simulink model "MCU_Simulation_Architecture"  (R2022b)
settings: Solver=FixedStepDiscrete  StartTime=0.0  StopTime=10  FixedStep=TimeSteps.ModelStep  RelTol=1e-6
PreLoadFcn:
  | addpath('tools');
  | addpath('tools\Config_UI');
  | addpath('tools\support');
  | addpath('tools\support\PlantModel');
  | addpath('tools\FMIKit_for_Simulink');
  | addpath('tools\SpeedCommand');
  | addpath('tools\SpeedCommand\exe');
  | addpath('tools\SpeedCommand\view');
  | addpath('tools\MciAPI');
  | addpath('tools\MciAPI\exe');
  | addpath('tools\MciAPI\exe\enums');
  | addpath('tools\Read_PDB_File');
  | addpath('tools\Read_PDB_File\exe');
  | addpath('tools\PILComm');
  | addpath('tools\PILComm\exe');
  | addpath('tools\CompileLink');
  | 
  | addpath('exe');
  | addpath('source');
  | addpath(genpath('plant_model'))
  | addpath(genpath('ParametersFiles'))
  | 
  | clear all;
  | 
  | try
  | FMIKit.initialize()
  | catch
  | display('FMI Kit Initialization Skipped');
  | end
  | 
  | Sim_Arch_Config_UI_App;
PostLoadFcn:
  | myws = get_param(gcs, 'modelworkspace');
  | myws.clear;
  | clear myws;
  | evalin('base', 'recompile_mcu_sim_arch = 1;');
  | updateModelWS(gcs);
  | 
  | variant_adc_out_mode = 0; % SIL Mode
  | 
  | ModelConfig_init_MCU_SimArch;
InitFcn:
  | if (evalin('base', 'exist(''smlarch_need_reset'') == 1'))
  |     msgbox('Reload Variables before Running');
  |     set_param(gcs, 'SimulationCommand', 'stop');
  | end
  | BusInit;
  | if(  (exist('SimArchUID')) && (strcmp(SimArchUID, 'a') == 1)  )
  |     updateModelWS(gcs);
  | end
  | useModelWS(gcs);
  | Simulink.sdi.close;
model workspace (MAT data in the model file):
  DC_Bus.Const_Vbus = 325
  InputCircuit.R_line = 0.8
  InputCircuit.L_line = 5e-05
  InputCircuit.C_buscap = 0.00022
  InputCircuit.R_diode = 0.068
  InputCircuit.R_buscap = 0.904
  InputCircuit.V_knee = 0.75
  InputCircuit.G_off = 1.25e-08
  InputCircuit.L_pfc = 0.0035
  InputCircuit.R_pfc = 0.45
  InputCircuit.Vr = 230
  InputCircuit.Vdc_i = 300
  InputCircuit.freq = 50
  InputCircuit.C1 = -0.200926
  InputCircuit.C2 = 1.64303
  InputCircuit.Cvolt = 0.00738585
  InputCircuit.Vcc = 3.3
  InputCircuit.ADCBit = 12
  InputCircuit.PGA_Gain = 1
  Mechanical.belt_ratio = 10
  Mechanical.JDrum = 0.0636792
  Mechanical.damp = 0.28
  Mechanical.m_unb = 0
  Mechanical.r_unb = 0.254
  Mechanical.M_D = 1
  Mechanical.M = 0.2
  Mechanical.R_Drum = 0.254
  Mechanical.R_J = 0.05
  Mechanical.CF = 0
  Motor.Electrical.Rs_a_Ref = 2.87
  Motor.Electrical.Rs_b_Ref = 2.87
  Motor.Electrical.Rs_c_Ref = 2.87
  Motor.Electrical.p_Pole_Pairs = 4
  Motor.Electrical.PM_Flux_f01 = 0.0845
  Motor.Electrical.PM_Flux_f02 = 0
  Motor.Electrical.PM_Flux_f03 = 0
  Motor.Electrical.PM_Flux_f04 = 0
  Motor.Electrical.PM_Flux_f05 = 0
  Motor.Electrical.PM_Flux_f06 = 0
  Motor.Electrical.PM_Flux_f07 = 0
  Motor.Electrical.PM_Flux_f08 = 0
  Motor.Electrical.PM_Flux_f09 = 0
  Motor.Electrical.PM_Flux_f10 = 0
  Motor.Electrical.PM_Flux_f11 = 0
  Motor.Electrical.PM_Flux_f12 = 0
  Motor.Electrical.PM_Flux_f13 = 0
  Motor.Electrical.ajust = 1.57
  Motor.Electrical.alpha_s = 0.004
  Motor.Mechanical.Jrotor = 0.000515
  Motor.Mechanical.B = 0
  Motor.Mechanical.Jadd = 0
  Motor.Mechanical.Rs_Temperature_Ref = 22
  Motor.Mechanical.PM_Temperature_Ref = 22
  Motor.Mechanical.TR = 11.4
  Motor.Power_Loss.Rot_Loss_Flag = 0
  Motor.Power_Loss.Rot_Loss_Speed0 = 0
  Motor.Power_Loss.Rot_Loss_Speed1 = 500
  Motor.Power_Loss.Rot_Loss_Speed2 = 3000
  Motor.Power_Loss.Rot_Loss_Speed3 = 4000
  Motor.Power_Loss.Rot_Loss_Speed4 = 5000
  Motor.Power_Loss.Rot_Loss_Speed5 = 7000
  Motor.Power_Loss.Rot_Loss_Speed6 = 12000
  Motor.Power_Loss.Rot_Loss_Speed7 = 18000
  Motor.Power_Loss.Rot_Loss_Power0 = 0
  Motor.Power_Loss.Rot_Loss_Power1 = 1
  Motor.Power_Loss.Rot_Loss_Power2 = 12
  Motor.Power_Loss.Rot_Loss_Power3 = 19
  Motor.Power_Loss.Rot_Loss_Power4 = 26
  Motor.Power_Loss.Rot_Loss_Power5 = 35
  Motor.Power_Loss.Rot_Loss_Power6 = 41
  Motor.Power_Loss.Rot_Loss_Power7 = 56
  Motor.Inductance_Variation.Ld_a0 = 0.02117
  Motor.Inductance_Variation.Ld_a1 = 0.02117
  Motor.Inductance_Variation.Ld_a2 = 0.02117
  Motor.Inductance_Variation.Ld_a3 = 0.02117
  Motor.Inductance_Variation.Ld_a4 = 0.02117
  Motor.Inductance_Variation.Ld_a5 = 0.02117
  Motor.Inductance_Variation.Ld_a6 = 0.02117
  Motor.Inductance_Variation.Ld_a7 = 0.02117
  Motor.Inductance_Variation.Lq_b0 = 0.02744
  Motor.Inductance_Variation.Lq_b1 = 0.02777
  Motor.Inductance_Variation.Lq_b2 = 0.02742
  Motor.Inductance_Variation.Lq_b3 = 0.02646
  Motor.Inductance_Variation.Lq_b4 = 0.02426
  Motor.Inductance_Variation.Lq_b5 = 0.02329
  Motor.Inductance_Variation.Lq_b6 = 0.02241
  Motor.Inductance_Variation.Lq_b7 = 0.02241
  Motor.Inductance_Variation.I_pk0 = 0
  Motor.Inductance_Variation.I_pk1 = 1
  Motor.Inductance_Variation.I_pk2 = 2
  Motor.Inductance_Variation.I_pk3 = 3
  Motor.Inductance_Variation.I_pk4 = 4
  Motor.Inductance_Variation.I_pk5 = 5
  Motor.Inductance_Variation.I_pk6 = 6
  Motor.Inductance_Variation.I_pk7 = 7
  Paths.complete_file_R = 'ParametersFiles\Board_Parameters\HVPS_230VPFC\WindyStripH40_AC230VPFC.xml'
  Paths.complete_file_M = 'ParametersFiles\Motor_Parameters\BPM\sBPM\BPM_Hefei_H27.xml'
  Paths.complete_file_mc = 'ParametersFiles\Mechanical_Parameters\HA\Mechanical_HA.xml'
  Paths.chosen_dir_M = 'ParametersFiles\Motor_Parameters\BPM\sBPM'
  Paths.Setting_File_Path = 'C:\Users\BEDNASA\Desktop\HA_sBPM_T95123402.bin'
  Paths.Root_Path = 'C:\Data\Nucleus_Dev\Windy_MCU_sBPM\source'
  Paths.Object_Path = ''
  Thermal.Tstator = 22
  Thermal.Trotor = 22
  TimeSteps.ModelStep = 6.25e-05
  TimeSteps.InputCircuitStep = 6.25e-05
  Variant_Input_Circuit = 4
  Variant_Motor = 4
  Variant_Motor_Control = 1
  Variant_Sensor = 0
  config.MCI_Sampling_Frequency = 'Set'
  config.rect_flag = 0
  config.const_dcbus_flag = 1
  config.Root_Path_flag = 'Source Selected'
  config.Motor_Control_Source = 'Set'
  config.Control_Layer = 'SIL'
  config.Fast_ADC_Initialization_Flag = 'Set'
  config.Skip_Motor_Moving_Handler_Flag = 'Set'
  config.BoardVariant = 'AC230VPFC'
  config.MotorVariant = 'BPM_Hefei_H27'
  config.MechanicalVariant = 'HA_Spin'
  config.Setting_File_Flag = 'Set'
undefined symbols (not defined in the file): sigbuilder_block, steps
CloseFcn:
  | rmpath('support');
  | rmpath('Compile Scripts');
  | rmpath(genpath('plant_models'))
  | rmpath(genpath('MciAPI'));
  | clc;
  | clear all;
settings Model: Creator=consul.marchionne  LastModifiedBy=BEDNASA
settings SolverCC: AlgebraicLoopSolver=TrustRegion
settings DataIOCC: LimitDataPoints=on  ReturnWorkspaceOutputs=off
settings OptimizationCC: LifeSpan=inf
settings DebuggingCC: SolverPrmCheckMsg=warning  UnconnectedInputMsg=warning  UnconnectedOutputMsg=warning  UnconnectedLineMsg=warning  SFUnexpectedBacktrackingDiag=warning  SFNoUnconditionalDefaultTransitionDiag=warning  SFExecutionAtInitializationDiag=none  SFMachineParentedDataDiag=warning  ArithmeticOperatorsInVariantConditions=warning
settings HardwareCC: ProdBitPerPointer=32  ProdBitPerSizeT=32  ProdBitPerPtrDiffT=32  ProdLargestAtomicFloat=None  ProdIntDivRoundTo=Undefined  ProdEndianess=Unspecified  ProdWordSize=32  ProdHWDeviceType=32-bit Generic
settings ModelReferenceCC: UpdateModelReferenceTargets=IfOutOfDate  ModelReferenceNumInstancesAllowed=Single  ModelReferenceMinAlgLoopOccurrences=on  PropagateSignalLabelsOutOfModel=off
settings SFSimCC: SimUseLocalCustomCode=off  CustomCodeUndefinedFunction=UseInterfaceOnly
settings RTWCC: RTWUseLocalCustomCode=off
settings CodeAppCC: StateflowObjectComments=on
settings GRTTargetCC: TargetLangStandard=C89/C90 (ANSI)
settings ConfigComp: CovMetricSettings=dw  CovSaveCumulativeToWorkspaceVar=on  CovSaveSingleToWorkspaceVar=on  CovExternalEMLEnable=off  CovSFcnEnable=off

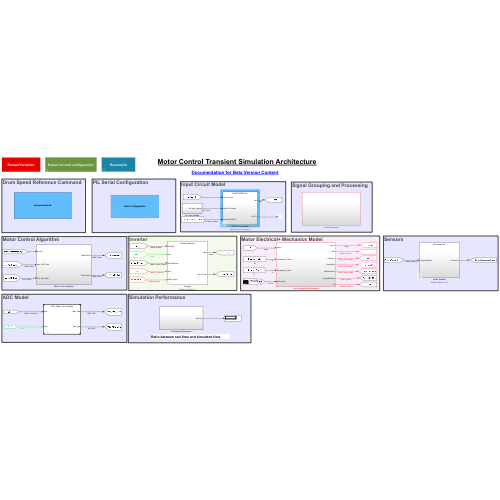
[thumbnail: Simulink's stored preview of the top-level diagram]
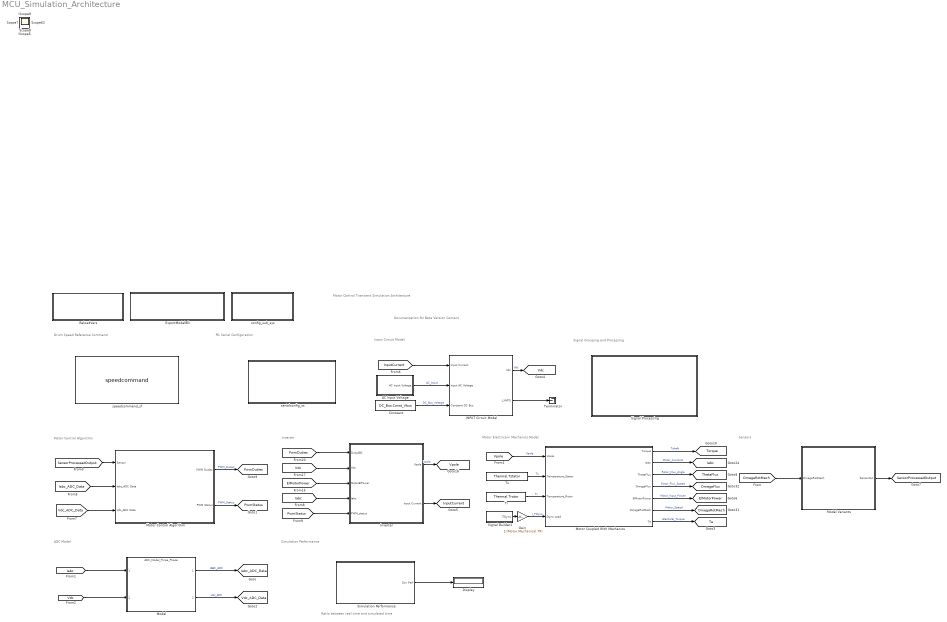
== system MCU_Simulation_Architecture ==
  note: Motor Control Transient Simulation Architecture
  note: Input Circuit Model
  note: Simulation Performance
  note: Ratio between real time and simulated time
  note: ADC Model
  note: Motor Electrical+ Mechanics Model
  note: Inverter
  note: Signal Grouping and Processing
  note: PIL Serial Configuration
  note: Motor Control Algorithm
  note: Sensors
  note: Drum Speed Reference Command
  note: Documentation for Beta Version Content
  AC Input Voltage : Subsystem
  Constant : Constant  Value=DC_Bus.Const_Vbus
  Display : Display
  ExportModelBlk : Subsystem  LoadFcn=|  mask{model_name=}
      | msk = Simulink.Mask.get(gcb);
      | bHandle = msk.getDialogControl('Control2');
      | bHandle.Enabled = 'on';
      | clear msk;
      | clear bHandle;
      mask prompts: model_name "Model's export name (no extension)"
      mask DialogControl Control2 Prompt: Export
      mask DialogControl Control2 Callback:
      | save_system('MCU_Simulation_Architecture');
      | if (strcmp(get_param(gcb, 'model_name'),'') == 1)
      |     msgbox('Must give a name to the model');
      | else
      |     exportSimArch(get_param(gcb, 'model_name'));
      | end
      mask Display: disp('Export current configuration');
  Gain : Gain  Gain=1/(Motor.Mechanical.TR)
  INPUT Circuit Model : Subsystem  Variant=on
      settings: AttributesFormatString=%<ActiveVariant>
  Inverter : Subsystem  Variant=on  mask(Inverter ideal){}
      mask help: Ideal model of 3-phase inverter
      settings: AttributesFormatString=%<ActiveVariant>
  Model : ModelReference  ModelNameDialog=ADC_Model_Three_Phase.slx  UsingDefaultArgumentValue=0,0,0,0,0,0,0,0,0,0,0,0  SimulationMode=Normal  ModelReferenceVersion=1.0  Gain_Iabc=InputCircuit.C1  Offset_Iabc=InputCircuit.C2  Vcc_Iabc=InputCircuit.Vcc  ADCBit_Iabc=InputCircuit.ADCBit  PGA_Gain_Iabc=1  Out_mode_Iabc=0  Gain_Vdc=InputCircuit.Cvolt  Offset_Vdc=0  Vcc_Vdc=InputCircuit.Vcc  ADCBit_Vdc=InputCircuit.ADCBit  PGA_Gain_Vdc=1  Out_mode_Vdc=0  SimulationMode=Normal
  Model Variants : Subsystem  Variant=on
      settings: AttributesFormatString=%<ActiveVariant>
  Motor Control Algorithm : Subsystem  SystemSampleTime=6.25e-5
  Motor Coupled With Mechanics : Subsystem  SystemSampleTime=0.000125
      settings: CopyFcn=|
      | blockname = gcb;
      |  linkstatus = lower(get_param(blockname,'LinkStatus'));
      | if strcmp(linkstatus,'resolved')
      |   set_param(gcb,'LinkStatus','none');
      | end
  ReloadVars : Subsystem
      settings: OpenFcn=|
      | evalin('base', 'clear smlarch_need_reset');
      | useModelWS(gcs);
      mask Display: disp('Reload Variables');
  Signal Builder1 : Subsystem  Tag=STV Subsys  LoadFcn=sigbuilder_block('load');  StartFcn=sigbuilder_block('start');  StopFcn=sigbuilder_block('stop');  ClipboardFcn=sigbuilder_block('clipboard');  mask(Sigbuilder block){tuvar=[0:10]}
      mask help: Simulink:masks:SigbuilderBlock_MD
      mask init:
      | if ~strcmp(get_param(bdroot(gcbh),'SimulationStatus'),'stopped') tuvar = sigbuilder_block('maskInit'); end
      settings: CopyFcn=sigbuilder_block('copy');  DeleteFcn=sigbuilder_block('delete');  ModelCloseFcn=sigbuilder_block('modelClose');  PreSaveFcn=sigbuilder_block('preSave');  PauseFcn=sigbuilder_block('pause');  ContinueFcn=sigbuilder_block('continue');  NameChangeFcn=sigbuilder_block('namechange');  OpenFcn=sigbuilder_block('open',[150 123 461.25 300 ]);  CloseFcn=sigbuilder_block('close');
      mask Display: plot(0, 0, 100, 100,[2, 2, 32, 32, 2], [68, 8, 8, 68, 68],[32, 2], [38, 38], [32, 19, 2],[53, 60, 44], [32, 17, 17, 2],[16, 16, 31, 31]);txt = getActiveGroup(gcbh);text(2, 100, txt,'verticalAlignment', 'top');
  Signal Processing : Subsystem
  Simulation Performance : Subsystem
  Terminator : Terminator
  Tr : Constant  Value=Thermal.Trotor
  Ts : Constant  Value=Thermal.Tstator
  config_sub_sys : Subsystem  TreatAsAtomicUnit=on  mask{mcu_recompile=on}
      mask prompts: mcu_recompile "Recompile"
      mask Display:
      | if (strcmp(get_param(gcb, 'mcu_recompile'),'off') == 1)
      |     disp('Do not Recompile');
      | else
      |     disp('Recompile');
      | end
  serialconfig_ss : Subsystem  mask{comdevtype=RS232, com_port=COM4, baudrate=57600}
      mask prompts: comdevtype "COM Type"; com_port "COM Port"
      mask TypeOptions comdevtype: RS232 | SPI
      mask Callback comdevtype:
      | maskStr = get_param(gcb,'comdevtype');
      | if strcmp(maskStr,'SPI')
      |     assignin('base', 'VARIANT_PIL_COMM', 2);
      | else
      |     assignin('base', 'VARIANT_PIL_COMM', 1);
      | end
      | clear maskStr;
      mask TypeOptions com_port: COM3 | COM4
      mask TypeOptions baudrate: 2400 | 4800 | 9600 | 19200 | 28800 | 38400 | 57600 | 115200 | 230400
      mask DialogControl ParameterGroupVar Prompt: RS232 Settings
      mask DialogControl rfrsh_button Prompt: Refresh Ports
      mask DialogControl rfrsh_button Callback:
      | devices = winqueryreg('name', 'HKEY_LOCAL_MACHINE', 'HARDWARE\DEVICEMAP\SERIALCOMM');
      | if (isempty(devices))
      |     com{1} = 'NONE';
      | else
      |     com = cell(1, length(devices));
      |    % h = waitbar(0,'Scanning Serial Ports...','Name','Scanning Serial Ports...');
      |     for i = 1:length(devices)
      |         com{i} = winqueryreg('HKEY_LOCAL_MACHINE', 'HARDWARE\DEVICEMAP\SERIALCOMM', devices{i});
      |     %    waitbar(i/length(devices),h);
      |     end
      | end
      | 
      | msk = Simulink.Mask.get(gcb);
      | p = msk.Parameters;
      | p(2).TypeOptions = com;
      | clear msk;
      | clear p;
      | clear com;
      | clear devices;
      mask Display: disp('Serial Configuration');
  speedcommand_sf : S-Function  InitFcn=|  StopFcn=|  FunctionName=speedcommand  Parameters=steps, Variant_Motor_Control  SFunctionDeploymentMode=off  EnableBusSupport=off
      InitFcn=|
      | transmission = evalin('base','Motor.Mechanical.TR');
      | if isempty(get_param(gcb,'UserData'))
      | steps = [];
      | else
      |     ud = get_param(gcb,'UserData');
      |     [pts,steps] = GenPlotCmds(ud.table);
      |     for i = 1:size(steps,1)
      |         steps(i,1) = steps(i,1) * transmission;
      |         steps(i,2) = steps(i,2) * transmission;
      |     end
      | end
      | clear transmission;
      | clear i;
      | clear ud;
      StopFcn=|
      | clear steps;
      | clear pts;
      settings: OpenFcn=SpeedCommandView;
  Scope{,2..12} (12 alike) : Scope
  tag scope: ElMotorPower=global, Iabc=global, Iabc_ADC_Data=global, InputCurrent=global, OmegaFlux=global, OmegaRotMech=global, PwmDuties=global, PwmStatus=global, SensorProcessedOutput=global, Te=global, ThetaFlux=global, Torque=global, Vdc=global, Vdc_ADC_Data=global, Vpole=global
  wires:
  Simulation Performance/1(Sim Perf) -> Display/1
  [Vpole] -> Motor Coupled With Mechanics/1(Vpole)  "Vpole"
  Motor Coupled With Mechanics/1(Torque) -> [Torque]  "Tshaft"
  Motor Coupled With Mechanics/2(Iabc) -> [Iabc]  "Motor_Currents"
  Motor Coupled With Mechanics/3(ThetaFlux) -> [ThetaFlux]  "Rotor_Flux_Angle"
  Motor Coupled With Mechanics/4(OmegaFlux) -> [OmegaFlux]  "Rotor_Flux_Speed"
  Motor Coupled With Mechanics/5(ElMotorPower) -> [ElMotorPower]  "Motor_Input_Power"
  Motor Coupled With Mechanics/6(OmegaRotMech) -> [OmegaRotMech]  "Motor_Speed"
  Motor Control Algorithm/1(PWM Duties) -> [PwmDuties]  "PWM_Duties"
  Motor Control Algorithm/2(PWM Status) -> [PwmStatus]  "PWM_Status"
  [SensorProcessedOutput] -> Motor Control Algorithm/1(Sensor)
  [Vdc] -> Model/2
  [Iabc] -> Model/1
  [Iabc_ADC_Data] -> Motor Control Algorithm/2(Iabc_ADC Data)
  Model/1 -> [Iabc_ADC_Data]  "IABC_ADC"
  Model/2 -> [Vdc_ADC_Data]  "Vdc_ADC"
  [Vdc_ADC_Data] -> Motor Control Algorithm/3(Vdc_ADC Data)
  Ts/1 -> Motor Coupled With Mechanics/2(Temperature_Stator)  "Ts"
  Tr/1 -> Motor Coupled With Mechanics/3(Temperature_Rotor)  "Tr"
  Gain/1 -> Motor Coupled With Mechanics/4(Dyno Load)  "i_TDyno"
  Signal Builder1/1(iTDyno) -> Gain/1
  Motor Coupled With Mechanics/7(Te) -> [Te]  "Electrical_Torque"
  [InputCurrent] -> INPUT Circuit Model/1(Input Current)
  AC Input Voltage/1(AC Input Voltage) -> INPUT Circuit Model/2(Input AC Voltage)  "AC_Input"
  Constant/1 -> INPUT Circuit Model/3(Constant DC Bus)  "DC_Bus_Voltage"
  INPUT Circuit Model/1(Vdc) -> [Vdc]  "Vdc"
  [PwmDuties] -> Inverter/1(DutyABC)
  [Vdc] -> Inverter/2(Vdc)
  [ElMotorPower] -> Inverter/3(MotorElPower)
  [Iabc] -> Inverter/4(Iabc)
  [PwmStatus] -> Inverter/5(PWM_status)
  Inverter/1(Vpole) -> [Vpole]  "Vpole"
  Inverter/2(Input Current) -> [InputCurrent]
  [OmegaRotMech] -> Model Variants/1(OmegaRotMech)
  Model Variants/1(SensorOut) -> [SensorProcessedOutput]
  INPUT Circuit Model/2(I_HVPS) -> Terminator/1

== system MCU_Simulation_Architecture/AC Input Voltage ==
  Sine Wave : Sin  Amplitude=InputCircuit.Vr*sqrt(2)  Frequency=InputCircuit.freq*2*pi
  AC Input Voltage : Outport  VectorParamsAs1DForOutWhenUnconnected=off
  wires:
  Sine Wave/1 -> AC Input Voltage/1

== system MCU_Simulation_Architecture/ExportModelBlk ==

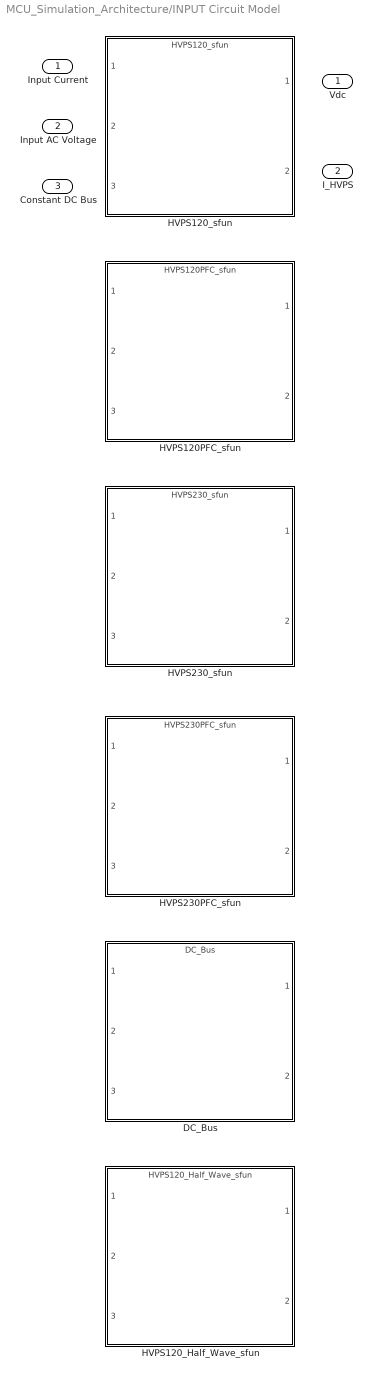
== system MCU_Simulation_Architecture/INPUT Circuit Model ==
  Input Current : Inport
  Input AC Voltage : Inport  Port=2
  Constant DC Bus : Inport  Port=3
  DC_Bus : ModelReference  ModelNameDialog=DC_Bus.slx  SimulationMode=Normal  VariantControl=Variant_Input_Circuit==5  ModelReferenceVersion=10.0
      settings: AttributesFormatString=%<ActiveVariant>
  HVPS120PFC_sfun : ModelReference  ModelNameDialog=HVPS120PFC_sfun.slx  SimulationMode=Normal  VariantControl=Variant_Input_Circuit==2  ModelReferenceVersion=10.4
      settings: AttributesFormatString=%<ActiveVariant>
  HVPS120_Half_Wave_sfun : ModelReference  ModelNameDialog=HVPS120_Half_Wave_sfun.slx  SimulationMode=Normal  VariantControl=Variant_Input_Circuit==6  ModelReferenceVersion=10.6
      settings: AttributesFormatString=%<ActiveVariant>
  HVPS120_sfun : ModelReference  ModelNameDialog=HVPS120_sfun.slx  SimulationMode=Normal  VariantControl=Variant_Input_Circuit==1  ModelReferenceVersion=10.8
      settings: AttributesFormatString=%<ActiveVariant>
  HVPS230PFC_sfun : ModelReference  ModelNameDialog=HVPS230PFC_sfun.slx  SimulationMode=Normal  VariantControl=Variant_Input_Circuit==4  ModelReferenceVersion=10.16
      settings: AttributesFormatString=%<ActiveVariant>
  HVPS230_sfun : ModelReference  ModelNameDialog=HVPS230_sfun.slx  SimulationMode=Normal  VariantControl=Variant_Input_Circuit==3  ModelReferenceVersion=10.3
      settings: AttributesFormatString=%<ActiveVariant>
  Vdc : Outport
  I_HVPS : Outport  Port=2

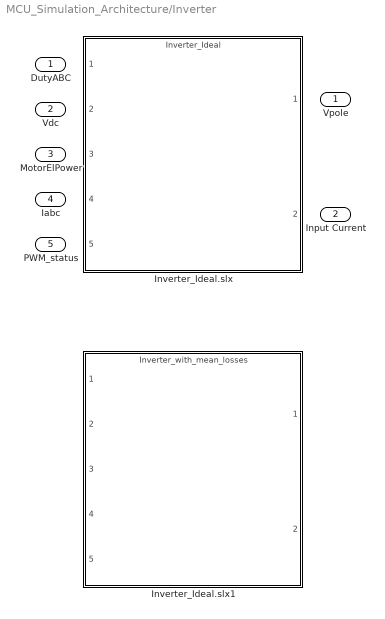
== system MCU_Simulation_Architecture/Inverter ==
  DutyABC : Inport  OutDataTypeStr=Bus: XabcBus
  Vdc : Inport  Port=2
  MotorElPower : Inport  Port=3
  Iabc : Inport  Port=4  OutDataTypeStr=Bus: XabcBus
  PWM_status : Inport  Port=5
  Inverter_Ideal.slx : ModelReference  ModelNameDialog=Inverter_Ideal.slx  SimulationMode=Normal  VariantControl=Variant_Inverter==1  OverrideUsingVariant=Variant1  ModelReferenceVersion=1.19  SimulationMode=Normal
      settings: AttributesFormatString=%<ActiveVariant>
  Inverter_Ideal.slx1 : ModelReference  ModelNameDialog=Inverter_with_mean_losses.slx  SimulationMode=Normal  VariantControl=Variant_Inverter==2  OverrideUsingVariant=Variant1  ModelReferenceVersion=10.27
      settings: AttributesFormatString=%<ActiveVariant>
  Vpole : Outport  OutDataTypeStr=Bus: XabcBus
  Input Current : Outport  Port=2

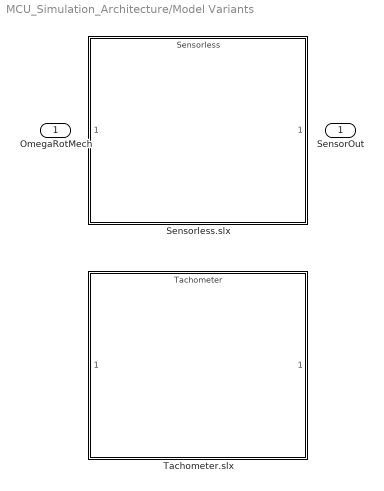
== system MCU_Simulation_Architecture/Model Variants ==
  OmegaRotMech : Inport
  Sensorless.slx : ModelReference  ModelNameDialog=Sensorless.slx  SimulationMode=Normal  VariantControl=Variant_Sensor == 0  ModelReferenceVersion=1.8
      settings: AttributesFormatString=%<ActiveVariant>
  Tachometer.slx : ModelReference  ModelNameDialog=Tachometer.slx  SimulationMode=Normal  VariantControl=Variant_Sensor == 1  ModelReferenceVersion=1.34
      settings: AttributesFormatString=%<ActiveVariant>
  SensorOut : Outport

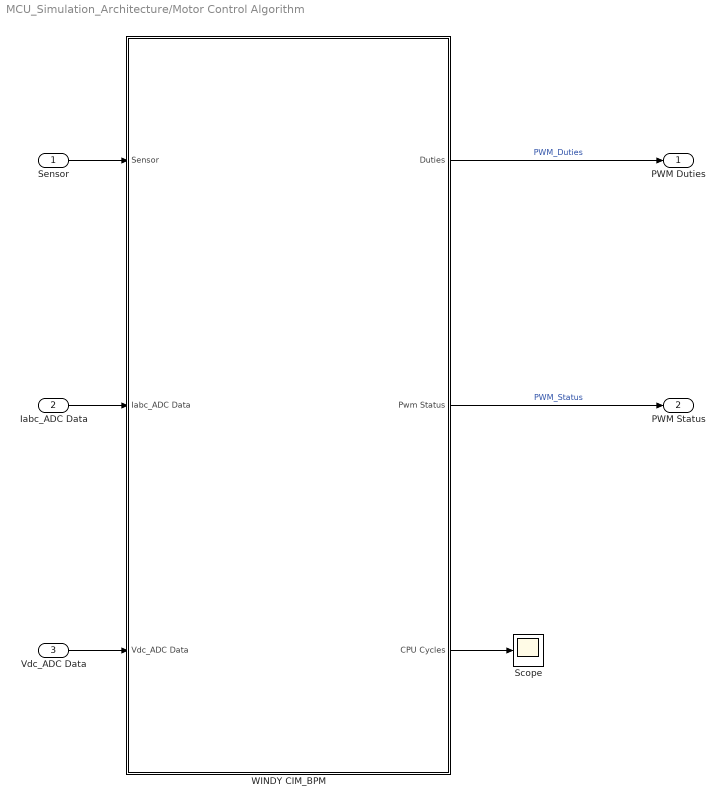
== system MCU_Simulation_Architecture/Motor Control Algorithm ==
  Sensor : Inport
  Iabc_ADC Data : Inport  Port=2
  Vdc_ADC Data : Inport  Port=3
  Scope : Scope
  WINDY CIM_BPM : Subsystem  Variant=on
  PWM Duties : Outport  VectorParamsAs1DForOutWhenUnconnected=off
  PWM Status : Outport  Port=2  VectorParamsAs1DForOutWhenUnconnected=off
  wires:
  WINDY CIM_BPM/1(Duties) -> PWM Duties/1  "PWM_Duties"
  WINDY CIM_BPM/2(Pwm Status) -> PWM Status/1  "PWM_Status"
  Sensor/1 -> WINDY CIM_BPM/1(Sensor)
  Iabc_ADC Data/1 -> WINDY CIM_BPM/2(Iabc_ADC Data)
  Vdc_ADC Data/1 -> WINDY CIM_BPM/3(Vdc_ADC Data)
  WINDY CIM_BPM/3(CPU Cycles) -> Scope/1

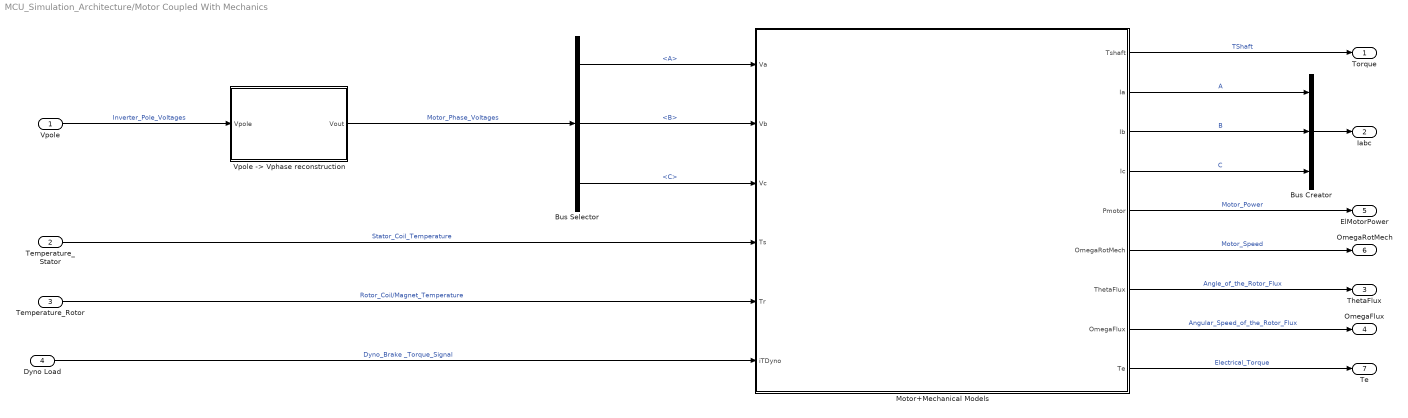
== system MCU_Simulation_Architecture/Motor Coupled With Mechanics ==
  Vpole : Inport  OutDataTypeStr=Bus: XabcBus
  Temperature_Stator : Inport  Port=2
  Temperature_Rotor : Inport  Port=3
  Dyno Load : Inport  Port=4
  Bus Creator : BusCreator  Inputs=3
  Bus Selector : BusSelector  OutputSignals=A,B,C
  Motor+Mechanical Models : Subsystem  Variant=on
      settings: AttributesFormatString=%<ActiveVariant>
  "Vpole -> Vphase reconstruction" : MATLAB Function  TreatAsAtomicUnit=on
  Torque : Outport  VectorParamsAs1DForOutWhenUnconnected=off
  Iabc : Outport  Port=2  OutDataTypeStr=Bus: XabcBus  VectorParamsAs1DForOutWhenUnconnected=off
  ThetaFlux : Outport  Port=3  VectorParamsAs1DForOutWhenUnconnected=off
  OmegaFlux : Outport  Port=4  VectorParamsAs1DForOutWhenUnconnected=off
  ElMotorPower : Outport  Port=5  VectorParamsAs1DForOutWhenUnconnected=off
  OmegaRotMech : Outport  Port=6  VectorParamsAs1DForOutWhenUnconnected=off
  Te : Outport  Port=7  VectorParamsAs1DForOutWhenUnconnected=off
  wires:
  Bus Creator/1 -> Iabc/1
  Vpole/1 -> "Vpole -> Vphase reconstruction"/1(Vpole)  "Inverter_Pole_Voltages"
  "Vpole -> Vphase reconstruction"/1(Vout) -> Bus Selector/1  "Motor_Phase_Voltages"
  Bus Selector/1 -> Motor+Mechanical Models/1(Va)  "<A>"
  Bus Selector/2 -> Motor+Mechanical Models/2(Vb)  "<B>"
  Bus Selector/3 -> Motor+Mechanical Models/3(Vc)  "<C>"
  Temperature_Stator/1 -> Motor+Mechanical Models/4(Ts)  "Stator_Coil_Temperature"
  Temperature_Rotor/1 -> Motor+Mechanical Models/5(Tr)  "Rotor_Coil/Magnet_Temperature"
  Dyno Load/1 -> Motor+Mechanical Models/6(iTDyno)  "Dyno_Brake _Torque_Signal"
  Motor+Mechanical Models/1(Tshaft) -> Torque/1  "TShaft"
  Motor+Mechanical Models/2(Ia) -> Bus Creator/1  "A"
  Motor+Mechanical Models/3(Ib) -> Bus Creator/2  "B"
  Motor+Mechanical Models/4(Ic) -> Bus Creator/3  "C"
  Motor+Mechanical Models/5(Pmotor) -> ElMotorPower/1  "Motor_Power"
  Motor+Mechanical Models/6(OmegaRotMech) -> OmegaRotMech/1  "Motor_Speed"
  Motor+Mechanical Models/7(ThetaFlux) -> ThetaFlux/1  "Angle_of_the_Rotor_Flux"
  Motor+Mechanical Models/8(OmegaFlux) -> OmegaFlux/1  "Angular_Speed_of_the_Rotor_Flux"
  Motor+Mechanical Models/9(Te) -> Te/1  "Electrical_Torque"

== system MCU_Simulation_Architecture/ReloadVars ==

== system MCU_Simulation_Architecture/Signal Builder1 ==
  Demux : Demux  Tag=STV Demux  Outputs=1
      settings: DisplayOption=none
  FromWs : FromWorkspace  Tag=STV FromWs  VariableName=tuvar
      SigBuilderData=|
      | common.afterFinalStr = 'Extrapolate'
      | common.sampleTime = 0
      | dataSet.timeRange = [0 30]
      | dataSet.name = 'Dyno_Load_Profile'
      | sbobj.Groups.Name = 'Dyno_Load_Profile'
      | sbobj.Groups.Signals.Name = 'iTDyno'
      | sbobj.Groups.Signals.XData = [0 0.8 4 20 28 30]
      | sbobj.Groups.Signals.YData = [0 0 0 0 0 0]
      | sbobj.Groups.TimeRange = [0 30]
  iTDyno : Outport  Tag=STV Outport  VectorParamsAs1DForOutWhenUnconnected=off
  wires:
  Demux/1 -> iTDyno/1
  FromWs/1 -> Demux/1

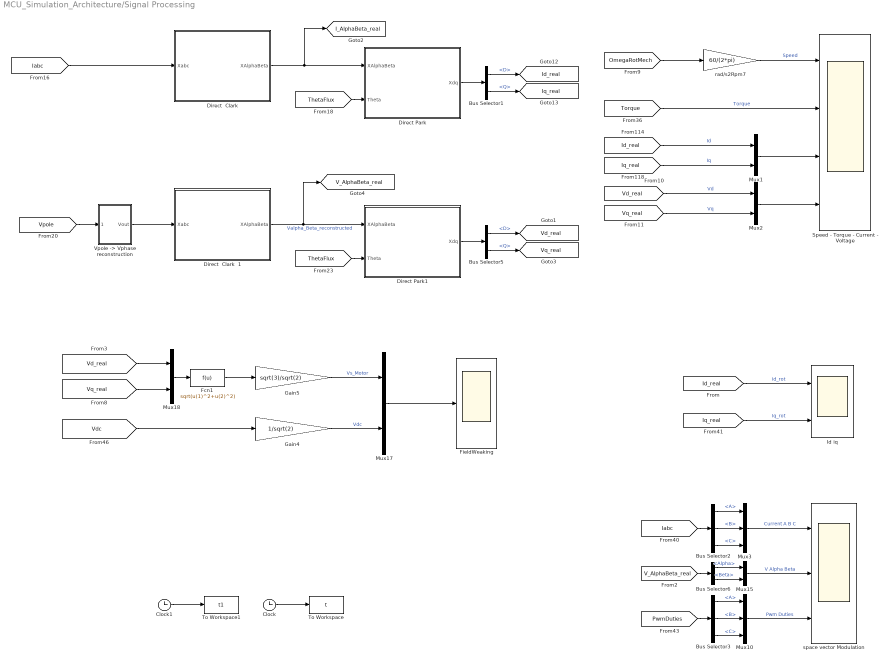
== system MCU_Simulation_Architecture/Signal Processing ==
  Bus Selector1 : BusSelector  OutputSignals=D,Q
  Bus Selector2 : BusSelector  OutputSignals=A,B,C
  Bus Selector3 : BusSelector  OutputSignals=A,B,C
  Bus Selector5 : BusSelector  OutputSignals=D,Q
  Bus Selector6 : BusSelector  OutputSignals=Alpha,Beta
  Clock : Clock
  Clock1 : Clock
  "Direct  Clark  " : MATLAB Function  TreatAsAtomicUnit=on  SystemSampleTime=SystemSampleTime  mask{SystemSampleTime=-1}
      mask prompts: SystemSampleTime "Simulink:blkprm_prompts:AllBlksSampleTime"
  Direct  Clark  1 : MATLAB Function  TreatAsAtomicUnit=on  SystemSampleTime=SystemSampleTime  mask{SystemSampleTime=-1}
      mask prompts: SystemSampleTime "Simulink:blkprm_prompts:AllBlksSampleTime"
  Direct Park : MATLAB Function  TreatAsAtomicUnit=on  SystemSampleTime=SystemSampleTime  mask{SystemSampleTime=-1}
      mask prompts: SystemSampleTime "Simulink:blkprm_prompts:AllBlksSampleTime"
  Direct Park1 : MATLAB Function  TreatAsAtomicUnit=on  SystemSampleTime=SystemSampleTime  mask{SystemSampleTime=-1}
      mask prompts: SystemSampleTime "Simulink:blkprm_prompts:AllBlksSampleTime"
  Fcn1 : Fcn  Expr=sqrt(u(1)^2+u(2)^2)
  "FieldWeaking " : Scope
  Gain4 : Gain  Gain=1/sqrt(2)
  Gain5 : Gain  Gain=sqrt(3)/sqrt(2)
  Id iq : Scope  NumInputPorts=2
  Mux{1..2,15,17..18} (5 alike) : Mux  Inputs=2
  Mux10 : Mux  Inputs=3
  Mux3 : Mux  Inputs=3
  Speed - Torque - Current - Voltage : Scope  NumInputPorts=4
  To Workspace : ToWorkspace  VariableName=t  SampleTime=-1
      settings: Save2DSignal=2-D array (concatenate along first dimension)
  To Workspace1 : ToWorkspace  VariableName=t1  SampleTime=-1
      settings: Save2DSignal=2-D array (concatenate along first dimension)
  "Vpole -> Vphase reconstruction" : MATLAB Function  TreatAsAtomicUnit=on
  rad/s2Rpm7 : Gain  Gain=60/(2*pi)
  space vector Modulation : Scope  NumInputPorts=3
  tag scope: I_AlphaBeta_real=global, Id_real=global, Iq_real=global, V_AlphaBeta_real=global, Vd_real=global, Vq_real=global
  wires:
  [OmegaRotMech] -> rad/s2Rpm7/1
  rad/s2Rpm7/1 -> Speed - Torque - Current - Voltage/1  "Speed"
  [Vq_real] -> Mux2/2  "Vq"
  [Id_real] -> Mux1/1  "Id"
  [Iabc] -> "Direct  Clark  "/1(Xabc)
  Direct Park/1(Xdq) -> Bus Selector1/1
  Bus Selector1/1 -> [Id_real]  "<D>"
  Bus Selector1/2 -> [Iq_real]  "<Q>"
  Fcn1/1 -> Gain5/1
  Mux18/1 -> Fcn1/1
  [Vd_real] -> Mux18/1
  [Vq_real] -> Mux18/2
  Mux17/1 -> "FieldWeaking "/1
  [Vdc] -> Gain4/1
  Bus Selector3/1 -> Mux10/1  "<A>"
  Bus Selector3/2 -> Mux10/2  "<B>"
  Bus Selector3/3 -> Mux10/3  "<C>"
  Mux10/1 -> space vector Modulation/3  "Pwm Duties"
  Bus Selector2/1 -> Mux3/1  "<A>"
  Bus Selector2/2 -> Mux3/2  "<B>"
  Bus Selector2/3 -> Mux3/3  "<C>"
  [Iabc] -> Bus Selector2/1
  [PwmDuties] -> Bus Selector3/1
  "Direct  Clark  "/1(XAlphaBeta) -> [I_AlphaBeta_real], Direct Park/1(XAlphaBeta)
  Clock/1 -> To Workspace/1
  Clock1/1 -> To Workspace1/1
  [Id_real] -> Id iq/1  "Id_rot"
  [Iq_real] -> Id iq/2  "Iq_rot"
  Gain4/1 -> Mux17/2  "Vdc"
  Gain5/1 -> Mux17/1  "Vs_Motor"
  Mux3/1 -> space vector Modulation/1  "Current A B C"
  [ThetaFlux] -> Direct Park/2(Theta)
  "Vpole -> Vphase reconstruction"/1(Vout) -> Direct  Clark  1/1(Xabc)
  [Vpole] -> "Vpole -> Vphase reconstruction"/1(Vpole)
  Direct  Clark  1/1(XAlphaBeta) -> Direct Park1/1(XAlphaBeta), [V_AlphaBeta_real]  "Valpha_Beta_reconstructed"
  [V_AlphaBeta_real] -> Bus Selector6/1
  Bus Selector6/1 -> Mux15/1  "<Alpha>"
  Bus Selector6/2 -> Mux15/2  "<Beta>"
  Mux15/1 -> space vector Modulation/2  "V Alpha Beta"
  Bus Selector5/2 -> [Vq_real]  "<Q>"
  Bus Selector5/1 -> [Vd_real]  "<D>"
  [ThetaFlux] -> Direct Park1/2(Theta)
  Direct Park1/1(Xdq) -> Bus Selector5/1
  [Iq_real] -> Mux1/2  "Iq"
  [Vd_real] -> Mux2/1  "Vd"
  [Torque] -> Speed - Torque - Current - Voltage/2  "Torque"
  Mux2/1 -> Speed - Torque - Current - Voltage/4
  Mux1/1 -> Speed - Torque - Current - Voltage/3

== system MCU_Simulation_Architecture/Simulation Performance ==
  Clock : Clock
  MATLAB Function : MATLAB Function  TreatAsAtomicUnit=on
  Sim Perf : Outport  VectorParamsAs1DForOutWhenUnconnected=off
  wires:
  MATLAB Function/1(y) -> Sim Perf/1
  Clock/1 -> MATLAB Function/1(t)

== system MCU_Simulation_Architecture/config_sub_sys ==

== system MCU_Simulation_Architecture/serialconfig_ss ==

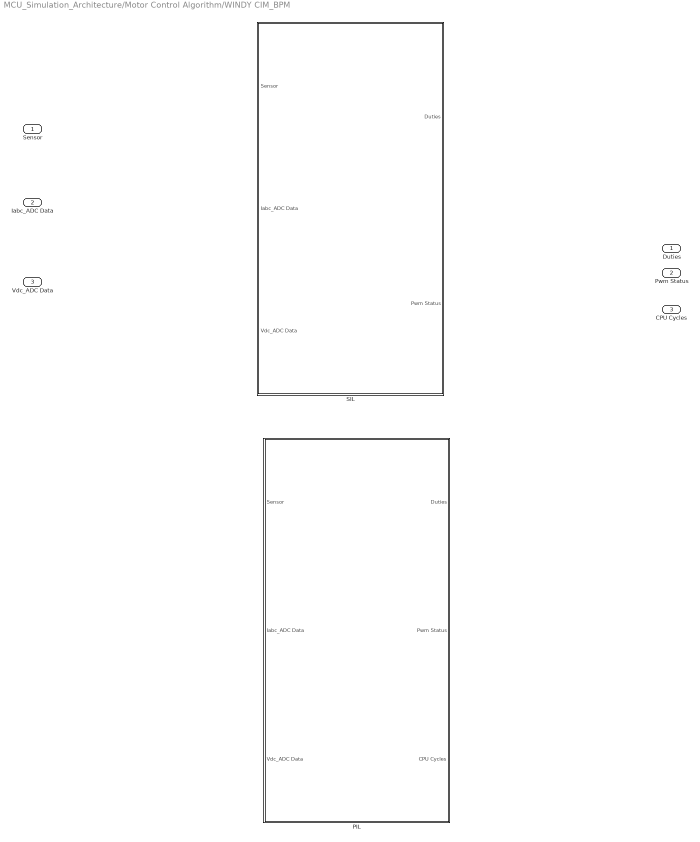
== system MCU_Simulation_Architecture/Motor Control Algorithm/WINDY CIM_BPM ==
  Sensor : Inport
  Iabc_ADC Data : Inport  Port=2
  Vdc_ADC Data : Inport  Port=3
  PIL : Subsystem  InitFcn=|  VariantControl=Variant_Motor_Control==2
      | Control_Layer=evalin('base','config.Control_Layer');
      | 
      | switch Control_Layer
      |    case 'MCI'
      | 
      |      Compile_Link_MCI(config.Root_Path_flag, Paths.Root_Path, config.Motor, Paths.Object_Path)
      | 
      | case 'MCU'
      |    
      |      Compile_Link_MCU(config.Root_Path_flag, Paths.Root_Path, config.Motor, Paths.Object_Path)
      | end
      | 
      | clear Control_Layer;
  SIL : Subsystem  VariantControl=Variant_Motor_Control==1
  Duties : Outport  VectorParamsAs1DForOutWhenUnconnected=off
  Pwm Status : Outport  Port=2  VectorParamsAs1DForOutWhenUnconnected=off
  CPU Cycles : Outport  Port=3  VectorParamsAs1DForOutWhenUnconnected=off

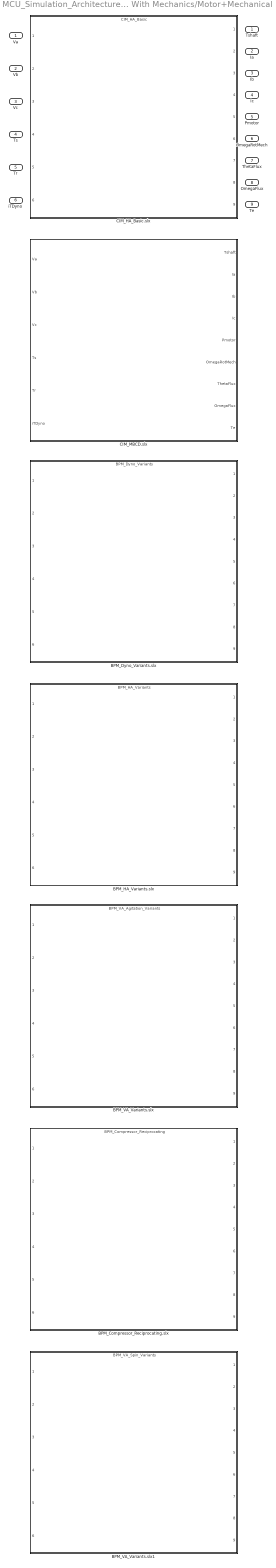
== system MCU_Simulation_Architecture/Motor Coupled With Mechanics/Motor+Mechanical Models ==
  Va : Inport
  Vb : Inport  Port=2
  Vc : Inport  Port=3
  Ts : Inport  Port=4
  Tr : Inport  Port=5
  iTDyno : Inport  Port=6
  BPM_Compressor_Reciprocating.slx : ModelReference  ModelNameDialog=BPM_Compressor_Reciprocating.slx  SimulationMode=Normal  VariantControl=Variant_Motor==8  ModelReferenceVersion=1.199
      settings: AttributesFormatString=%<ActiveVariant>
  BPM_Dyno_Variants.slx : ModelReference  ModelNameDialog=BPM_Dyno_Variants.slx  SimulationMode=Normal  VariantControl=Variant_Motor==3  ModelReferenceVersion=10.11
      settings: AttributesFormatString=%<ActiveVariant>
  BPM_HA_Variants.slx : ModelReference  ModelNameDialog=BPM_HA_Variants.slx  SimulationMode=Normal  VariantControl=Variant_Motor==4  ModelReferenceVersion=10.9
      settings: AttributesFormatString=%<ActiveVariant>
  BPM_VA_Variants.slx : ModelReference  ModelNameDialog=BPM_VA_Agitation_Variants.slx  SimulationMode=Normal  VariantControl=Variant_Motor==5  ModelReferenceVersion=10.9
      settings: AttributesFormatString=%<ActiveVariant>
  BPM_VA_Variants.slx1 : ModelReference  ModelNameDialog=BPM_VA_Spin_Variants.slx  VariantControl=Variant_Motor==6  ModelReferenceVersion=10.4
      settings: AttributesFormatString=%<ActiveVariant>
  CIM_HA_Basic.slx : ModelReference  ModelNameDialog=CIM_HA_Basic.slx  SimulationMode=Normal  VariantControl=Variant_Motor==1  ModelReferenceVersion=1.20
      settings: AttributesFormatString=%<ActiveVariant>
  CIM_MBCD.slx : Subsystem  TreatAsAtomicUnit=on  VariantControl=Variant_Motor==2
  Tshaft : Outport
  Ia : Outport  Port=2
  Ib : Outport  Port=3
  Ic : Outport  Port=4
  Pmotor : Outport  Port=5
  OmegaRotMech : Outport  Port=6
  ThetaFlux : Outport  Port=7
  OmegaFlux : Outport  Port=8
  Te : Outport  Port=9

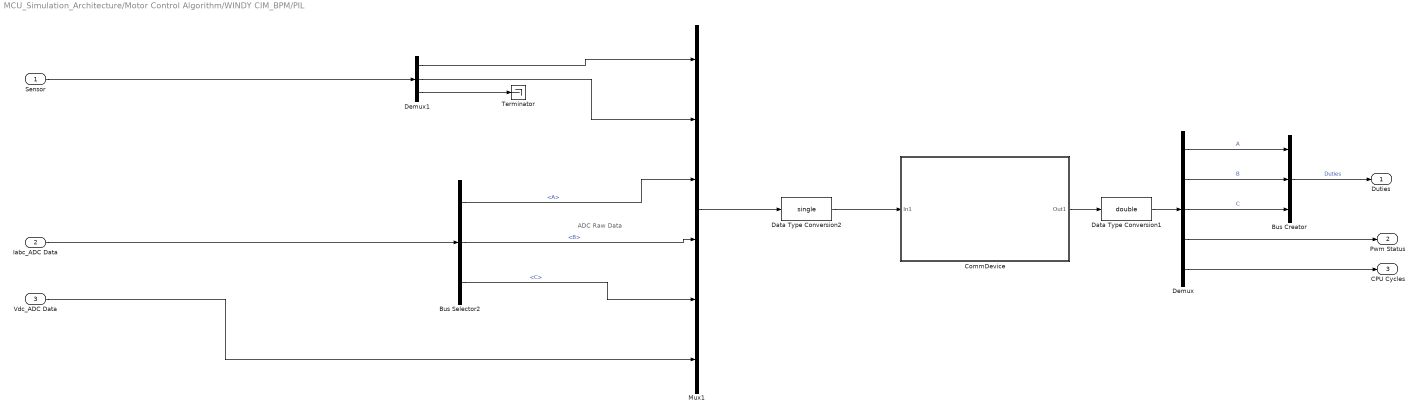
== system MCU_Simulation_Architecture/Motor Control Algorithm/WINDY CIM_BPM/PIL ==
  note: ADC Raw Data
  Sensor : Inport
  Iabc_ADC Data : Inport  Port=2
  Vdc_ADC Data : Inport  Port=3
  Bus Creator : BusCreator  Inputs=3
  Bus Selector2 : BusSelector  OutputSignals=A,B,C
  CommDevice : Subsystem  Variant=on  VariantControl=Variant1
  Data Type Conversion1 : DataTypeConversion  OutDataTypeStr=double  SaturateOnIntegerOverflow=off  RndMeth=Floor
  Data Type Conversion2 : DataTypeConversion  OutDataTypeStr=single  SaturateOnIntegerOverflow=off  RndMeth=Floor
  Demux : Demux  Outputs=5
  Demux1 : Demux  Outputs=3
  Mux1 : Mux  Inputs=6
  Terminator : Terminator
  Duties : Outport  VectorParamsAs1DForOutWhenUnconnected=off
  Pwm Status : Outport  Port=2  VectorParamsAs1DForOutWhenUnconnected=off
  CPU Cycles : Outport  Port=3  VectorParamsAs1DForOutWhenUnconnected=off
  wires:
  Bus Creator/1 -> Duties/1  "Duties"
  Bus Selector2/2 -> Mux1/4  "<B>"
  Bus Selector2/1 -> Mux1/3  "<A>"
  Bus Selector2/3 -> Mux1/5  "<C>"
  Vdc_ADC Data/1 -> Mux1/6
  Iabc_ADC Data/1 -> Bus Selector2/1
  Sensor/1 -> Demux1/1
  Demux1/3 -> Terminator/1
  Demux1/1 -> Mux1/1
  Demux1/2 -> Mux1/2
  Mux1/1 -> Data Type Conversion2/1
  Data Type Conversion2/1 -> CommDevice/1("In1 ")
  Data Type Conversion1/1 -> Demux/1
  Demux/4 -> Pwm Status/1
  Demux/1 -> Bus Creator/1  "A"
  Demux/2 -> Bus Creator/2  "B"
  Demux/3 -> Bus Creator/3  "C"
  CommDevice/1(" Out1") -> Data Type Conversion1/1
  Demux/5 -> CPU Cycles/1

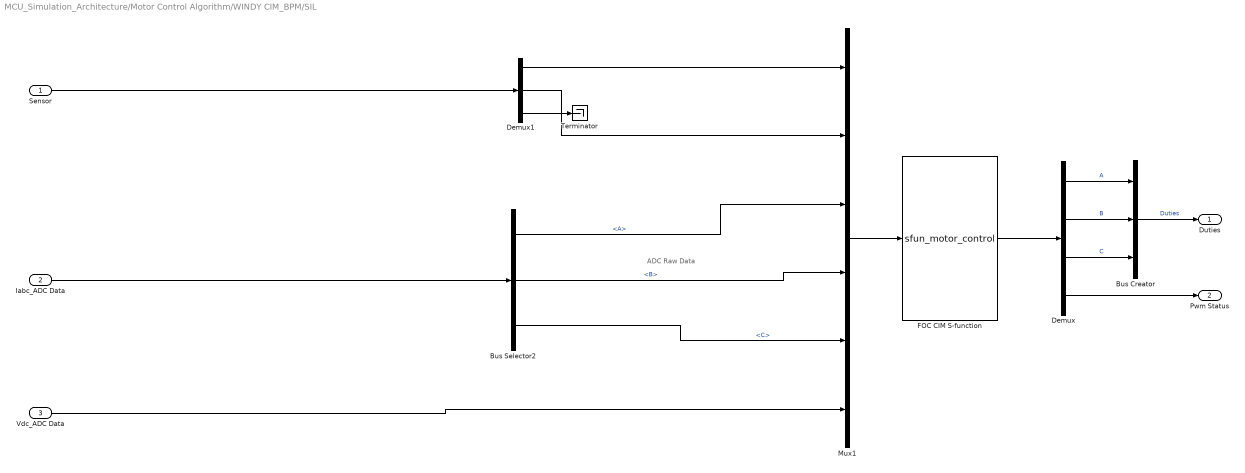
== system MCU_Simulation_Architecture/Motor Control Algorithm/WINDY CIM_BPM/SIL ==
  note: ADC Raw Data
  Sensor : Inport
  Iabc_ADC Data : Inport  Port=2
  Vdc_ADC Data : Inport  Port=3
  Bus Creator : BusCreator  Inputs=3
  Bus Selector2 : BusSelector  OutputSignals=A,B,C
  Demux : Demux
  Demux1 : Demux  Outputs=3
  "FOC CIM S-function " : S-Function  InitFcn=|  StopFcn=clear CompileStruct;  FunctionName=sfun_motor_control  Parameters=TimeSteps.ModelStep,Paths.Setting_File_Path  SFunctionDeploymentMode=off  EnableBusSupport=off
      | clear mex;
      | CompileStruct.Root_Path_flag=config.Root_Path_flag;
      | CompileStruct.Root_Path=Paths.Root_Path;
      | CompileStruct.Object_Path=Paths.Object_Path;
      | CompileStruct.Fast_ADC_Initialization_Flag=config.Fast_ADC_Initialization_Flag;
      | CompileStruct.Skip_Motor_Moving_Handler_Flag=config.Skip_Motor_Moving_Handler_Flag;
      | CompileStruct.Setting_File_Flag=config.Setting_File_Flag;
      | 
      | if ( (strcmp(get_param('MCU_Simulation_Architecture/config_sub_sys', 'mcu_recompile'), 'on') == 1) || (exist('SimArchUID')==0) || ( strcmp(SimArchUID, 'a') == 0 ) )
      |     Compile_Link_SimArch(CompileStruct);
      |     assignin('base', 'SimArchUID', 'a');
      | end
  Mux1 : Mux  Inputs=6
  Terminator : Terminator
  Duties : Outport  VectorParamsAs1DForOutWhenUnconnected=off
  Pwm Status : Outport  Port=2  VectorParamsAs1DForOutWhenUnconnected=off
  wires:
  Bus Selector2/2 -> Mux1/4  "<B>"
  "FOC CIM S-function "/1 -> Demux/1
  Bus Selector2/1 -> Mux1/3  "<A>"
  Bus Selector2/3 -> Mux1/5  "<C>"
  Vdc_ADC Data/1 -> Mux1/6
  Bus Creator/1 -> Duties/1  "Duties"
  Iabc_ADC Data/1 -> Bus Selector2/1
  Mux1/1 -> "FOC CIM S-function "/1
  Demux1/1 -> Mux1/1
  Demux1/2 -> Mux1/2
  Demux1/3 -> Terminator/1
  Sensor/1 -> Demux1/1
  Demux/1 -> Bus Creator/1  "A"
  Demux/2 -> Bus Creator/2  "B"
  Demux/3 -> Bus Creator/3  "C"
  Demux/4 -> Pwm Status/1

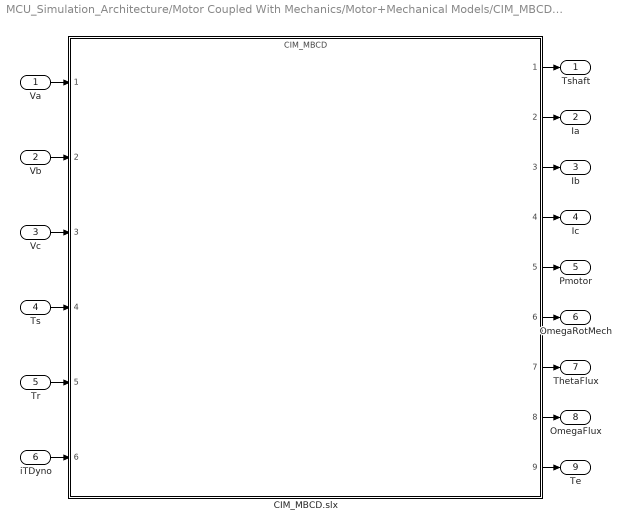
== system MCU_Simulation_Architecture/Motor Coupled With Mechanics/Motor+Mechanical Models/CIM_MBCD.slx ==
  Va : Inport
  Vb : Inport  Port=2
  Vc : Inport  Port=3
  Ts : Inport  Port=4
  Tr : Inport  Port=5
  iTDyno : Inport  Port=6
  CIM_MBCD.slx : ModelReference  ModelNameDialog=CIM_MBCD.slx  SimulationMode=Normal  ModelReferenceVersion=1.70
      settings: AttributesFormatString=%<ActiveVariant>
  Tshaft : Outport
  Ia : Outport  Port=2
  Ib : Outport  Port=3
  Ic : Outport  Port=4
  Pmotor : Outport  Port=5
  OmegaRotMech : Outport  Port=6
  ThetaFlux : Outport  Port=7
  OmegaFlux : Outport  Port=8
  Te : Outport  Port=9
  wires:
  CIM_MBCD.slx/7 -> ThetaFlux/1
  CIM_MBCD.slx/9 -> Te/1
  CIM_MBCD.slx/2 -> Ia/1
  CIM_MBCD.slx/5 -> Pmotor/1
  Tr/1 -> CIM_MBCD.slx/5
  iTDyno/1 -> CIM_MBCD.slx/6
  CIM_MBCD.slx/4 -> Ic/1
  CIM_MBCD.slx/3 -> Ib/1
  CIM_MBCD.slx/8 -> OmegaFlux/1
  CIM_MBCD.slx/1 -> Tshaft/1
  Va/1 -> CIM_MBCD.slx/1
  CIM_MBCD.slx/6 -> OmegaRotMech/1
  Vc/1 -> CIM_MBCD.slx/3
  Ts/1 -> CIM_MBCD.slx/4
  Vb/1 -> CIM_MBCD.slx/2

== system MCU_Simulation_Architecture/Motor Control Algorithm/WINDY CIM_BPM/PIL/CommDevice ==
  "In1 " : Inport
  RS232 : Subsystem  VariantControl=VARIANT_PIL_COMM == 1
  SPI : Subsystem  VariantControl=VARIANT_PIL_COMM == 2
  " Out1" : Outport  VectorParamsAs1DForOutWhenUnconnected=off

== system MCU_Simulation_Architecture/Motor Control Algorithm/WINDY CIM_BPM/PIL/CommDevice/RS232 ==
  In1 : Inport
  PIL_Comm : S-Function  InitFcn=|  FunctionName=serial_sf  Parameters=get_param([bdroot '/serialconfig_ss'], 'com_port'), get_param([bdroot '/serialconfig_ss'], 'baudrate'), steps  SFunctionDeploymentMode=off  EnableBusSupport=off
      | transmission = evalin('base','Motor.Mechanical.TR');
      | spd_blk = [bdroot '/speedcommand_sf']
      | if isempty(get_param(spd_blk,'UserData'))
      | steps = [];
      | else
      |     ud = get_param(spd_blk,'UserData');
      |     [pts,steps] = GenPlotCmds(ud.table);
      |     for i = 1:size(steps,1)
      |         steps(i,1) = steps(i,1) * transmission;
      |         steps(i,2) = steps(i,2) * transmission;
      |     end
      | end
      mask Display:
      | port_label('input', 1, 'Sim Inputs')
      | port_label('output', 1, 'Sim Outputs')
  Out1 : Outport  VectorParamsAs1DForOutWhenUnconnected=off
  wires:
  PIL_Comm/1 -> Out1/1
  In1/1 -> PIL_Comm/1

== system MCU_Simulation_Architecture/Motor Control Algorithm/WINDY CIM_BPM/PIL/CommDevice/SPI ==
  "In1 " : Inport
  S-Function : S-Function  InitFcn=|  FunctionName=cheetah_sf  Parameters=steps  SFunctionDeploymentMode=off  EnableBusSupport=off
      | transmission = evalin('base','Motor.Mechanical.TR');
      | spd_blk = [bdroot '/speedcommand_sf']
      | if isempty(get_param(spd_blk,'UserData'))
      | steps = [];
      | else
      |     ud = get_param(spd_blk,'UserData');
      |     [pts,steps] = GenPlotCmds(ud.table);
      |     for i = 1:size(steps,1)
      |         steps(i,1) = steps(i,1) * transmission;
      |         steps(i,2) = steps(i,2) * transmission;
      |     end
      | end
  " Out1" : Outport  VectorParamsAs1DForOutWhenUnconnected=off
  wires:
  "In1 "/1 -> S-Function/1
  S-Function/1 -> " Out1"/1

== matlab function MCU_Simulation_Architecture/Signal Processing/Direct  Clark  1 ==
  data: XAlphaBeta output Bus: XAlphaBetaBus; Xabc input Bus: XabcBus
function XAlphaBeta = DirectClark(Xabc)

XAlphaBeta.Alpha = Xabc.A;
XAlphaBeta.Beta =  sqrt(3)/3*(Xabc.A+2*Xabc.B);

== matlab function MCU_Simulation_Architecture/Signal Processing/Direct  Clark   ==
  data: XAlphaBeta output Bus: XAlphaBetaBus; Xabc input Bus: XabcBus
function XAlphaBeta = DirectClark(Xabc)

XAlphaBeta.Alpha = Xabc.A;
XAlphaBeta.Beta =  sqrt(3)/3*(Xabc.A+2*Xabc.B);

== matlab function MCU_Simulation_Architecture/Motor Coupled With Mechanics/Vpole -> Vphase reconstruction ==
  data: Vpole input Bus: XabcBus size=1; Vout output Bus: XabcBus
function Vout   = Vrec2(Vpole)

Va = Vpole.A;
Vb = Vpole.B;
Vc = Vpole.C;

Vn = (Va + Vb + Vc)/3;

Vphase.A = Va - Vn;
Vphase.B = Vb - Vn;
Vphase.C = Vc - Vn;

Vline.A = Va - Vb;  % Vab
Vline.B = Vb - Vc;  % Vbc
Vline.C = Vc - Va;  % Vca

Vout = Vphase;
end

== matlab function MCU_Simulation_Architecture/Simulation Performance/MATLAB Function ==
  data: t input; y output
function y = fcn(t)

persistent t_elaps tval sim_steps t_start t_end
coder.extrinsic('toc') 
coder.extrinsic('tic')
steps_start = 100;%10000;
steps_end = 500;%50000;

if isempty(tval)
    sim_steps = 0;
    tval = uint64(0);
    t_elaps = 0;
    t_start = 0;
    t_end = 0;
end
    
sim_steps = sim_steps +1;

if (sim_steps == steps_start)
    tval = tic;
    t_start = t;
     
end
if (sim_steps == steps_end)
    t_elaps = toc(tval);
    t_end = t;
end
 
if (t_elaps == 0)
    y = 0;
else
    y = t_elaps/(t_end-t_start);
 end

== matlab function MCU_Simulation_Architecture/Signal Processing/Direct Park ==
  data: XAlphaBeta input Bus: XAlphaBetaBus; Xdq output Bus: XdqBus; Theta input
function Xdq = DirectPark(XAlphaBeta,Theta)

Xdq.D  =  XAlphaBeta.Alpha*cos(Theta) + XAlphaBeta.Beta*sin(Theta);
Xdq.Q  = -XAlphaBeta.Alpha*sin(Theta) + XAlphaBeta.Beta*cos(Theta);

== matlab function MCU_Simulation_Architecture/Signal Processing/Direct Park1 ==
  data: XAlphaBeta input Bus: XAlphaBetaBus; Xdq output Bus: XdqBus; Theta input
function Xdq = DirectPark(XAlphaBeta,Theta)

Xdq.D  =  XAlphaBeta.Alpha*cos(Theta) + XAlphaBeta.Beta*sin(Theta);
Xdq.Q  = -XAlphaBeta.Alpha*sin(Theta) + XAlphaBeta.Beta*cos(Theta);

== matlab function MCU_Simulation_Architecture/Signal Processing/Vpole -> Vphase reconstruction ==
  data: Vpole input Bus: XabcBus size=1; Vout output Bus: XabcBus
function Vout   = Vrec2(Vpole)

Va = Vpole.A;
Vb = Vpole.B;
Vc = Vpole.C;

Vn = (Va + Vb + Vc)/3;

Vphase.A = Va - Vn;
Vphase.B = Vb - Vn;
Vphase.C = Vc - Vn;

Vline.A = Va - Vb;  % Vab
Vline.B = Vb - Vc;  % Vbc
Vline.C = Vc - Va;  % Vca

Vout = Vphase;
end
